simulink model "NCMS_AltMis_항공대"  (R2022a)
settings: Solver=FixedStepAuto  StartTime=0.0  StopTime=inf  FixedStep=SampleTime  RelTol=1e-3
InitFcn:
  | NCMS_AltMis_Init;
values from neighbouring files (symbols this model uses):
  Kdpr = 0.004    [NCMS_AltMis_Init_항공대.m]
  Kdrr = 0.004    [NCMS_AltMis_Init_항공대.m]
  Kdvz = 0.0254    [NCMS_AltMis_Init_항공대.m]
  Kdyr = 0.0298    [NCMS_AltMis_Init_항공대.m]
  Kipr = 0.1    [NCMS_AltMis_Init_항공대.m]
  Kirr = 0.1    [NCMS_AltMis_Init_항공대.m]
  Kivx = 0.0728/g    (= 0.00742099898063)    [NCMS_AltMis_Init_항공대.m]
  Kivy = 0.0728/g    (= 0.00742099898063)    [NCMS_AltMis_Init_항공대.m]
  Kivz = 0.6304    [NCMS_AltMis_Init_항공대.m]
  Kix = 0.02    [NCMS_AltMis_Init_항공대.m]
  Kiyaxis = 0.02    [NCMS_AltMis_Init_항공대.m]
  Kiyr = 0.7395    [NCMS_AltMis_Init_항공대.m]
  Kiz = 0.09    [NCMS_AltMis_Init_항공대.m]
  Kpp = 3.3894    [NCMS_AltMis_Init_항공대.m]
  Kppr = 0.1    [NCMS_AltMis_Init_항공대.m]
  Kpr = 3.3894    [NCMS_AltMis_Init_항공대.m]
  Kprr = 0.1    [NCMS_AltMis_Init_항공대.m]
  Kpvx = 2.1109/g    (= 0.215178389399)    [NCMS_AltMis_Init_항공대.m]
  Kpvy = 2.1109/g    (= 0.215178389399)    [NCMS_AltMis_Init_항공대.m]
  Kpvz = 0.3191    [NCMS_AltMis_Init_항공대.m]
  Kpx = 1    [NCMS_AltMis_Init_항공대.m]
  Kpy = 3.3894    [NCMS_AltMis_Init_항공대.m]
  Kpyaxis = 1    [NCMS_AltMis_Init_항공대.m]
  Kpyr = 0.3744    [NCMS_AltMis_Init_항공대.m]
  Kpz = 2.4    [NCMS_AltMis_Init_항공대.m]
  LAND_PRES_VEL = 0.2    [NCMS_AltMis_Init_항공대.m]
  MAX_CONTROL_ANGLE_PITCH = 30*pi/180    (= 0.523598775598)    [Init_FLIGHT_Hexacopter.m]    (also in NCMS_AltMis_Init_항공대.m = 0.349065850399)
  MAX_CONTROL_ANGLE_RATE_PITCH = 360*pi/180    (= 6.28318530718)    [Init_FLIGHT_Hexacopter.m]    (also in NCMS_AltMis_Init_항공대.m)
  MAX_CONTROL_ANGLE_RATE_ROLL = 360*pi/180    (= 6.28318530718)    [Init_FLIGHT_Hexacopter.m]    (also in NCMS_AltMis_Init_항공대.m)
  MAX_CONTROL_ANGLE_RATE_Y = 120*pi/180    (= 2.09439510239)    [Init_FLIGHT_Hexacopter.m]    (also in NCMS_AltMis_Init_항공대.m)
  MAX_CONTROL_ANGLE_ROLL = 30*pi/180    (= 0.523598775598)    [Init_FLIGHT_Hexacopter.m]    (also in NCMS_AltMis_Init_항공대.m = 0.349065850399)
  MAX_CONTROL_VELOCITY_XY = 1.5    [Init_FLIGHT_Hexacopter.m]    (also in NCMS_AltMis_Init_항공대.m)
  MAX_CONTROL_VELOCITY_Z = 1    [Init_FLIGHT_Hexacopter.m]    (also in NCMS_AltMis_Init_항공대.m)
  Npr = 50    [NCMS_AltMis_Init_항공대.m]
  Nrr = 50    [NCMS_AltMis_Init_항공대.m]
  Nvz = Npr    (= 50)    [NCMS_AltMis_Init_항공대.m]
  Nyr = 50    [NCMS_AltMis_Init_항공대.m]
  SampleTime = 1/250    (= 0.004)    [Init_FLIGHT_Hexacopter.m]    (also in NCMS_AltMis_Init_항공대.m = 0.01)
  THR_HOVER = 0.6085    [NCMS_AltMis_Init_항공대.m]
  THR_IDLE = 0.2    [NCMS_AltMis_Init_항공대.m]
undefined symbols (not defined in the file or in its folder): dev, Kdz, Main, Nz, pwm_output0
libraries: slpidlib x15, simulink x9, px4Sensorslib x3, px4uORBlib x3, uavalgslib x2, px4lib x1
(part 1 of 3)
settings Model: ExtModeTrigDuration=10  Creator=user  LastModifiedBy=ParkSeungWoo
settings SolverCC: PositivePriorityOrder=on
settings OptimizationCC: EnhancedBackFolding=on  PassReuseOutputArgsAs=Individual arguments  ZeroExternalMemoryAtStartup=off  ZeroInternalMemoryAtStartup=off  MaxStackSize=64  OptimizeBlockOrder=speed  DifferentSizesBufferReuse=on  OptimizationCustomize=off  EfficientTunableParamExpr=on
settings DebuggingCC: ParameterTunabilityLossMsg=error  UnconnectedInputMsg=warning  UnconnectedOutputMsg=warning  UnconnectedLineMsg=warning
settings HardwareCC: ProdBitPerPointer=32  ProdBitPerSizeT=32  ProdBitPerPtrDiffT=32  ProdLargestAtomicInteger=Long  ProdLargestAtomicFloat=Double  ProdWordSize=32  ProdLongLongMode=on  ProdHWDeviceType=ARM Compatible->ARM Cortex
settings SFSimCC: MATLABDynamicMemAlloc=off  SimTargetLang=C++
settings RTWCC: SystemTargetFile=ert.tlc  HardwareBoard=PX4 Pixhawk 4  TLCOptions="-aInlineSetEventsForThisBaseRateFcn=TLC_FALSE -aSuppressMultiTaskScheduler=TLC_FALSE  -aRateBasedStepFcn=0"  TemplateMakefile=ert_default_tmf  Toolchain=GNU Tools for PX4 Autopilots  TargetLang=C++  DLArmComputeVersion=19.05
settings CodeAppCC: ForceParamTrailComments=on  IgnoreCustomStorageClasses=off  OperatorAnnotations=on  SimulinkDataObjDesc=on  SFDataObjDesc=on  InsertBlockDesc=on
settings ERTTargetCC: MatFileLogging=on  ExtModeTransport=3  ExtModeStaticAlloc=on  ExtModeStaticAllocSize=1024  ExtModeMexFile=ext_xcp  ExtModeIntrfLevel=Level2 - Open

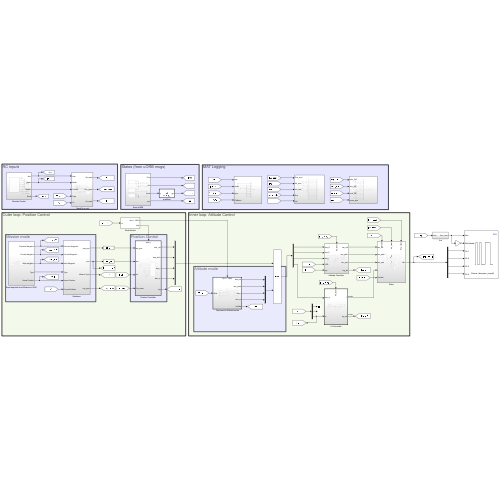
[thumbnail: Simulink's stored preview of the top-level diagram]
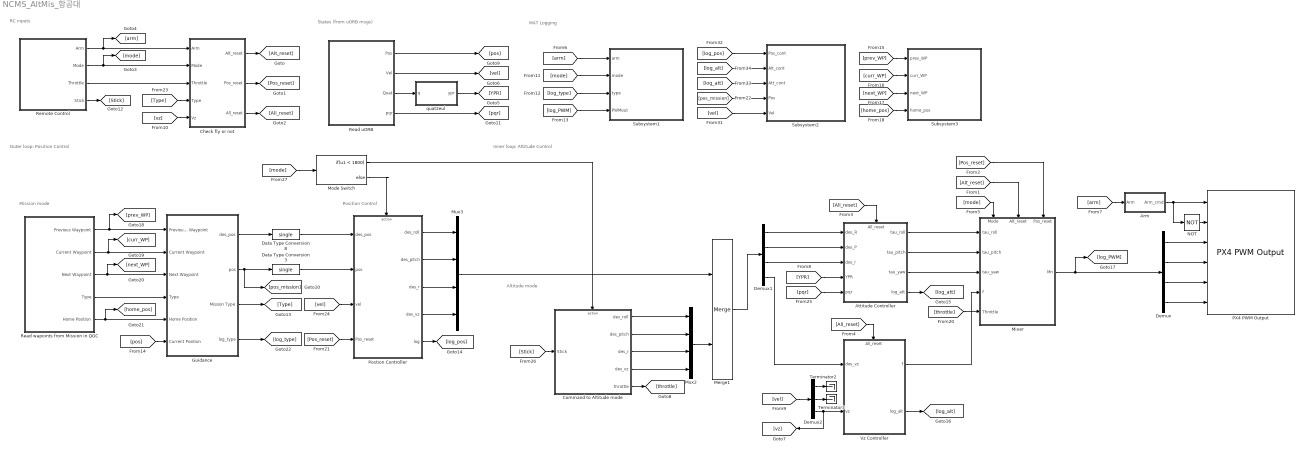
== system NCMS_AltMis_항공대 ==
  note: MAT Logging
  note: States (from uORB msgs)
  note: RC inputs
  note: Outer loop: Position Control
  note: Mission mode
  note: Inner loop: Attitude Control
  note: Altitude mode
  note: Position Control
  Arm : Subsystem
  Attitude Controller : Subsystem
      settings: PortSchema="{\"entries\":[{\"content\":{\"sides\":[{\"content\":{\"connectorIds\":[\"In1\",\"In2\",\"In3\",\"In4\",\"In5\"]},\"type\":\"ConnectorPlacement.EquallySpacedRectSide\",\"uuid\":\"77bb8164-b871-4593-8031-335c6110c17c\"},{\"content\":{\"connectorIds\":[\"Out1\",\"Out2\",\"Out3\",\"Out4\"],\"side\":\"RIGHT\"},\"type\":\"ConnectorPlacement.EquallySpacedRectSide\",\"uuid\":\"f99d9e85-7cc9-4d0a-ad5d-789571e28028\"},{\"content\":{\"connectorIds\":[\"In6\"],\"side\":\"TOP\"},\"type\":\"ConnectorPlacement.EquallySpacedRectSide\",\"uuid\":\"174eb658-0f52-43c7-ba1a-1a337b4835ca\"}]},\"type\":\"ConnectorPlacement.EquallySpacedConnector\",\"uuid\":\"7932b1f4-42ae-4dcf-8815-0888db42261d\"}],\"packageUris\":[\"http://schema.mathworks.com/mf0/Connector/R2020b\"],\"version\":\"1.0\"}"
  Check fly or not : Subsystem
  Command to Altitude mode : Subsystem  TreatAsAtomicUnit=on
  Data Type Conversion3 : DataTypeConversion  OutDataTypeStr=single  SaturateOnIntegerOverflow=off  RndMeth=Floor
  Data Type Conversion8 : DataTypeConversion  OutDataTypeStr=single  SaturateOnIntegerOverflow=off  RndMeth=Floor
  Demux : Demux
  Demux1 : Demux
  Demux2 : Demux  Outputs=3
  Guidance : Subsystem
  Merge1 : Merge
  Mixer : Subsystem
      settings: PortSchema="{\"entries\":[{\"content\":{\"sides\":[{\"content\":{\"connectorIds\":[\"In1\",\"In2\",\"In3\",\"In4\",\"In5\"]},\"type\":\"ConnectorPlacement.EquallySpacedRectSide\",\"uuid\":\"058a1e3b-c324-4fa3-8465-0a7a3d8b0c1a\"},{\"content\":{\"connectorIds\":[\"Out1\"],\"side\":\"RIGHT\"},\"type\":\"ConnectorPlacement.EquallySpacedRectSide\",\"uuid\":\"ff1c26dd-92d4-4453-a7b4-224d07c62cb4\"},{\"content\":{\"connectorIds\":[\"In6\",\"In7\",\"In8\"],\"side\":\"TOP\"},\"type\":\"ConnectorPlacement.EquallySpacedRectSide\",\"uuid\":\"9bc4c9d9-536a-4d54-a641-00bc48245afe\"}]},\"type\":\"ConnectorPlacement.EquallySpacedConnector\",\"uuid\":\"86048a90-d386-4461-986e-b57c6ef8ec17\"}],\"packageUris\":[\"http://schema.mathworks.com/mf0/Connector/R2020b\"],\"version\":\"1.0\"}"
  Mode Switch : If  IfExpression=u1 < 1800
  Mux2 : Mux
  Mux3 : Mux
  NOT : Logic  Operator=NOT  IconShape=distinctive  AllPortsSameDT=off  OutDataTypeStr=boolean
  PX4 PWM Output : px4lib/PX4 PWM Output  pwmDevice=Main (/dev/pwm_output0)  pwmChannel1_=on  pwmChannel2_=on  pwmChannel3_=on  pwmChannel4_=on  pwmChannel5_=off  pwmChannel6_=off  pwmChannel7_=off  pwmChannel8_=off  forceTerminateFailsafe=off  outputErrorStatus=off
      settings: SourceProductBaseCode=PX4AUTOPILOTS
  Postion Controller : Subsystem
  Read uORB : Subsystem
  Read wapoints from Mission in QGC : Subsystem
  Remote Control : Subsystem
  Subsystem1 : Subsystem
  Subsystem2 : Subsystem
  Subsystem3 : Subsystem
  Terminator2 : Terminator
  Terminator3 : Terminator
  Vz Controller : Subsystem  TreatAsAtomicUnit=on
      settings: PortSchema="{\"entries\":[{\"content\":{\"sides\":[{\"content\":{\"connectorIds\":[\"In1\",\"In2\"]},\"type\":\"ConnectorPlacement.EquallySpacedRectSide\",\"uuid\":\"343d190f-1f89-45cd-8068-8c2f27ac01d9\"},{\"content\":{\"connectorIds\":[\"Out1\",\"Out2\"],\"side\":\"RIGHT\"},\"type\":\"ConnectorPlacement.EquallySpacedRectSide\",\"uuid\":\"f56c4d57-5cdb-41f3-bf2e-c6d595243432\"},{\"content\":{\"connectorIds\":[\"In3\"],\"side\":\"TOP\"},\"type\":\"ConnectorPlacement.EquallySpacedRectSide\",\"uuid\":\"16744f99-c08a-4b46-9015-9ea58d319995\"}]},\"type\":\"ConnectorPlacement.EquallySpacedConnector\",\"uuid\":\"48685039-fe1b-4520-bbd0-43ddf02d7910\"}],\"packageUris\":[\"http://schema.mathworks.com/mf0/Connector/R2020b\"],\"version\":\"1.0\"}"
  quat2eul : MATLAB Function  TreatAsAtomicUnit=on
  wires:
  Demux/1 -> PX4 PWM Output/3
  Demux/2 -> PX4 PWM Output/4
  Demux/3 -> PX4 PWM Output/5
  Demux/4 -> PX4 PWM Output/6
  NOT/1 -> PX4 PWM Output/2
  Read uORB/3(Quat) -> quat2eul/1(q)
  Demux1/1 -> Attitude Controller/1(des_R)
  Demux1/2 -> Attitude Controller/2(des_P)
  Attitude Controller/1(tau_roll) -> Mixer/1(tau_roll)
  Attitude Controller/2(tau_pitch) -> Mixer/2(tau_pitch)
  Arm/1(Arm_cmd) -> NOT/1, PX4 PWM Output/1
  Demux1/3 -> Attitude Controller/3(des_r)
  Attitude Controller/3(tau_yaw) -> Mixer/3(tau_yaw)
  Demux2/2 -> Terminator3/1
  Demux2/1 -> Terminator2/1
  Vz Controller/1(f) -> Mixer/4(f)
  Demux2/3 -> Vz Controller/2(vz), [vz]
  Read uORB/2(Vel) -> [vel]
  Demux1/4 -> Vz Controller/1(des_vz)
  Mux2/1 -> Merge1/2
  Command to Altitude mode/3(des_r) -> Mux2/3
  Command to Altitude mode/2(des_pitch) -> Mux2/2
  Command to Altitude mode/1(des_roll) -> Mux2/1
  Command to Altitude mode/4(des_vz) -> Mux2/4
  Remote Control/4(Stick) -> [Stick]
  Postion Controller/2(des_pitch) -> Mux3/2
  Postion Controller/3(des_r) -> Mux3/3
  Postion Controller/1(des_roll) -> Mux3/1
  Mux3/1 -> Merge1/1
  Remote Control/2(Mode) -> [mode], Check fly or not/2(Mode)
  Remote Control/1(Arm) -> [arm], Check fly or not/1(Arm)
  Guidance/1(des_pos) -> Data Type Conversion8/1
  Read uORB/1(Pos) -> [pos]
  Postion Controller/4(des_vz) -> Mux3/4
  Data Type Conversion8/1 -> Postion Controller/1(des_pos)
  Data Type Conversion3/1 -> Postion Controller/2(pos)
  Merge1/1 -> Demux1/1
  Guidance/3(Mission Type) -> [Type]
  Check fly or not/1(Alt_reset) -> [Alt_reset]
  [Alt_reset] -> Mixer/7(Alt_reset)
  Check fly or not/2(Pos_reset) -> [Pos_reset]
  [Pos_reset] -> Mixer/8(Pos_reset)
  Check fly or not/3(All_reset) -> [All_reset]
  [All_reset] -> Attitude Controller/6(All_reset)
  [All_reset] -> Vz Controller/3(All_reset)
  [mode] -> Mixer/6(Mode)
  [arm] -> Arm/1(Arm)
  quat2eul/1(ypr) -> [YPR]
  [YPR] -> Attitude Controller/4(YPR)
  [vel] -> Demux2/1
  [vz] -> Check fly or not/5(Vz)
  [throttle] -> Mixer/5(Throttle)
  Command to Altitude mode/5(throttle) -> [throttle]
  [Pos_reset] -> Postion Controller/4(Pos_reset)
  Guidance/2(pos) -> [pos_mission], Data Type Conversion3/1
  [Type] -> Check fly or not/4(Type)
  Mode Switch/2 -> Postion Controller/Action
  Mode Switch/1 -> Command to Altitude mode/Action
  [vel] -> Postion Controller/3(vel)
  Read uORB/4(pqr) -> [pqr]
  [Stick] -> Command to Altitude mode/1(Stick)
  Remote Control/3(Throttle) -> Check fly or not/3(Throttle)
  [mode] -> Mode Switch/1
  Postion Controller/5(log) -> [log_pos]
  Attitude Controller/4(log_att) -> [log_att]
  Vz Controller/2(log_alt) -> [log_alt]
  Mixer/1(Mn) -> [log_PWM], Demux/1
  [arm] -> Subsystem1/1(arm)
  [mode] -> Subsystem1/2(mode)
  [log_type] -> Subsystem1/3(type)
  [log_PWM] -> Subsystem1/4(PWMout)
  [pos] -> Guidance/6(Current Position)
  Read wapoints from Mission in QGC/2(Current Waypoint) -> [curr_WP], Guidance/2(Current Waypoint)
  Read wapoints from Mission in QGC/3(Next Waypoint) -> [next_WP], Guidance/3(Next Waypoint)
  Read wapoints from Mission in QGC/4(Type) -> Guidance/4(Type)
  Read wapoints from Mission in QGC/5(Home Position) -> [home_pos], Guidance/5(Home Position)
  [pqr] -> Attitude Controller/5(pqr)
  [vel] -> Subsystem2/5(Vel)
  [pos_mission] -> Subsystem2/4(Pos)
  [log_att] -> Subsystem2/3(Att_cont)
  [log_alt] -> Subsystem2/2(Alt_cont)
  [log_pos] -> Subsystem2/1(Pos_cont)
  [home_pos] -> Subsystem3/4(home_pos)
  [next_WP] -> Subsystem3/3(next_WP)
  [curr_WP] -> Subsystem3/2(curr_WP)
  [prev_WP] -> Subsystem3/1(prev_WP)
  Guidance/4(log_type) -> [log_type]
  Read wapoints from Mission in QGC/1(Previous Waypoint) -> [prev_WP], Guidance/1(Previous Waypoint)

== system NCMS_AltMis_항공대/Arm ==
  Arm : Inport
  Compare To Constant3 : simulink/Logic and Bit Operations/Compare To Constant  relop=>=  const=uint16(1800)  OutDataTypeStr=boolean
  Arm_cmd : Outport  VectorParamsAs1DForOutWhenUnconnected=off
  wires:
  Arm/1 -> Compare To Constant3/1
  Compare To Constant3/1 -> Arm_cmd/1

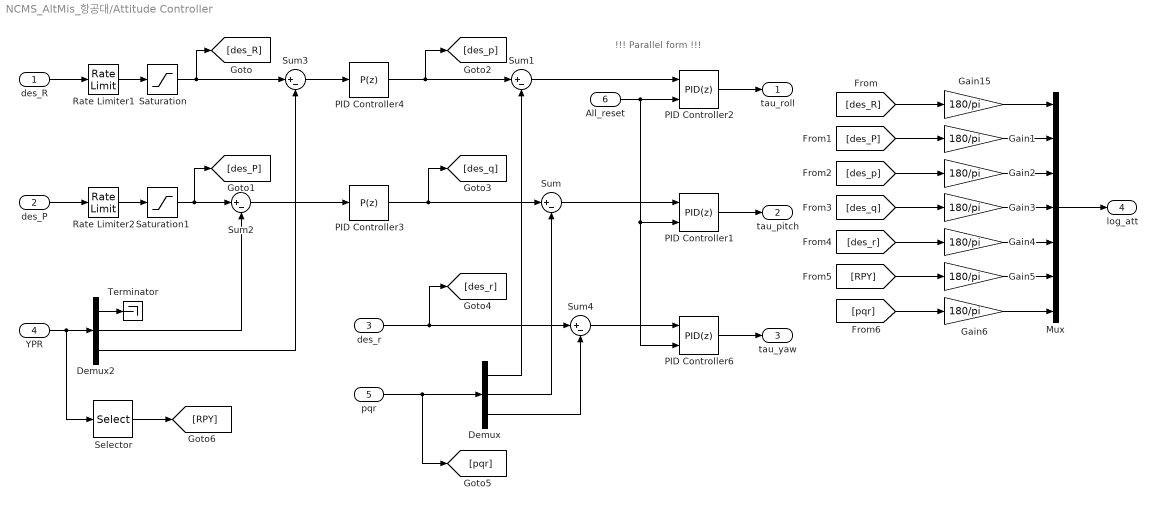
== system NCMS_AltMis_항공대/Attitude Controller ==
  note: !!! Parallel form !!!
  des_R : Inport
  des_P : Inport  Port=2
  des_r : Inport  Port=3
  YPR : Inport  Port=4
  pqr : Inport  Port=5
  All_reset : Inport  Port=6
  Demux : Demux  Outputs=3
  Demux2 : Demux  Outputs=3
  Gain{1..6,15} (7 alike) : Gain  Gain=180/pi
  Mux : Mux  Inputs=7
  PID Controller1 : slpidlib/PID Controller  Controller=PID  Form=Parallel  TimeDomain=Discrete-time  UseExternalTs=off  SampleTime=SampleTime  IntegratorMethod=Forward Euler  FilterMethod=Forward Euler  ControllerParametersSource=internal  P=Kppr  I=Kipr  UseKiTs=off  D=Kdpr  N=Npr  UseFilter=on  TunerSelectOption=Transfer Function Based (PID Tuner App)  InitialConditionSource=internal  InitialConditionForIntegrator=0  InitialConditionForFilter=0  DifferentiatorICPrevScaledInput=0  ExternalReset=either  TrackingMode=off  Kt=1  LimitOutput=on  SatLimitsSource=internal  UpperSaturationLimit=0.2  LowerSaturationLimit=-0.2  LinearizeAsGain=on  AntiWindupMode=clamping  Kb=1  POutMin=[]  POutMax=[]  IOutMin=[]  IOutMax=[]  DOutMin=[]  DOutMax=[]  NOutMin=[]  NOutMax=[]  SumOutMin=[]  SumOutMax=[]  SaturationOutMin=[]  SaturationOutMax=[]  PParamMin=[]  PParamMax=[]  IParamMin=[]  IParamMax=[]  DParamMin=[]  DParamMax=[]  NParamMin=[]  NParamMax=[]  KbParamMin=[]  KbParamMax=[]  KtParamMin=[]  KtParamMax=[]  KbOutMin=[]  KbOutMax=[]  KtOutMin=[]  KtOutMax=[]  IntegratorOutMin=[]  IntegratorOutMax=[]  FilterOutMin=[]  FilterOutMax=[]  SumI1OutMin=[]  SumI1OutMax=[]  SumI2OutMin=[]  SumI2OutMax=[]  SumI3OutMin=[]  SumI3OutMax=[]  SumI4OutMin=[]  SumI4OutMax=[]  SumDOutMin=[]  SumDOutMax=[]  DifferentiatorOutMin=[]  DifferentiatorOutMax=[]  FilterDiffOutCoefMin=[]  FilterDiffOutCoefMax=[]  ReciprocalOutMin=[]  ReciprocalOutMax=[]  SumDenOutMin=[]  SumDenOutMax=[]  SumNumOutMin=[]  SumNumOutMax=[]  DivideOutMin=[]  DivideOutMax=[]  UdiffTsProdOutMin=[]  UdiffTsProdOutMax=[]  NTsProdOutMin=[]  NTsProdOutMax=[]  UintegralTsProdOutMin=[]  UintegralTsProdOutMax=[]  UngainTsProdOutMin=[]  UngainTsProdOutMax=[]  IntegratorContinuousStateAttributes=''  IntegratorStateMustResolveToSignalObject=off  IntegratorRTWStateStorageClass=Auto  FilterContinuousStateAttributes=''  FilterStateMustResolveToSignalObject=off  FilterRTWStateStorageClass=Auto  ParallelPVariant=InternalParameters  IdealPVariant=Disabled  IVariant=InternalParameters  DVariant=InternalParameters  IntegratorVariant=Discrete  SatVariant=Enabled  AWVariant=DiscClampingParallel  PCopyVariant=Disabled  TRVariant=Disabled  FdbkBlocksVariant=Forward  IdealPFdbkVariant=Disabled  SatFdbkVariant=Disabled  DerivativeFilterVariant=ForwardEulerFilter  NVariant=InternalParameters  NCopyVariant=Disabled  FilterICVariant=InternalICsFilter  IntegratorICVariant=InternalICs  ExternalResetVariant=ExternalReset  TRSumVariant=Passthrough  SumFdbkVariant=Disabled  SumVariant=Sum_PID  TsampFilterVariant=InternalTs  TsampNgainVariant=Passthrough  TsampIntegralVariant=Passthrough  ExternalSaturationOutDataTypeStr=Inherit: Same as second input  aMode=0
  PID Controller2 : slpidlib/PID Controller  Controller=PID  Form=Parallel  TimeDomain=Discrete-time  UseExternalTs=off  SampleTime=SampleTime  IntegratorMethod=Forward Euler  FilterMethod=Forward Euler  ControllerParametersSource=internal  P=Kprr  I=Kirr  UseKiTs=off  D=Kdrr  N=Nrr  UseFilter=on  TunerSelectOption=Transfer Function Based (PID Tuner App)  InitialConditionSource=internal  InitialConditionForIntegrator=0  InitialConditionForFilter=0  DifferentiatorICPrevScaledInput=0  ExternalReset=either  TrackingMode=off  Kt=1  LimitOutput=on  SatLimitsSource=internal  UpperSaturationLimit=0.2  LowerSaturationLimit=-0.2  LinearizeAsGain=on  AntiWindupMode=clamping  Kb=1  POutMin=[]  POutMax=[]  IOutMin=[]  IOutMax=[]  DOutMin=[]  DOutMax=[]  NOutMin=[]  NOutMax=[]  SumOutMin=[]  SumOutMax=[]  SaturationOutMin=[]  SaturationOutMax=[]  PParamMin=[]  PParamMax=[]  IParamMin=[]  IParamMax=[]  DParamMin=[]  DParamMax=[]  NParamMin=[]  NParamMax=[]  KbParamMin=[]  KbParamMax=[]  KtParamMin=[]  KtParamMax=[]  KbOutMin=[]  KbOutMax=[]  KtOutMin=[]  KtOutMax=[]  IntegratorOutMin=[]  IntegratorOutMax=[]  FilterOutMin=[]  FilterOutMax=[]  SumI1OutMin=[]  SumI1OutMax=[]  SumI2OutMin=[]  SumI2OutMax=[]  SumI3OutMin=[]  SumI3OutMax=[]  SumI4OutMin=[]  SumI4OutMax=[]  SumDOutMin=[]  SumDOutMax=[]  DifferentiatorOutMin=[]  DifferentiatorOutMax=[]  FilterDiffOutCoefMin=[]  FilterDiffOutCoefMax=[]  ReciprocalOutMin=[]  ReciprocalOutMax=[]  SumDenOutMin=[]  SumDenOutMax=[]  SumNumOutMin=[]  SumNumOutMax=[]  DivideOutMin=[]  DivideOutMax=[]  UdiffTsProdOutMin=[]  UdiffTsProdOutMax=[]  NTsProdOutMin=[]  NTsProdOutMax=[]  UintegralTsProdOutMin=[]  UintegralTsProdOutMax=[]  UngainTsProdOutMin=[]  UngainTsProdOutMax=[]  IntegratorContinuousStateAttributes=''  IntegratorStateMustResolveToSignalObject=off  IntegratorRTWStateStorageClass=Auto  FilterContinuousStateAttributes=''  FilterStateMustResolveToSignalObject=off  FilterRTWStateStorageClass=Auto  ParallelPVariant=InternalParameters  IdealPVariant=Disabled  IVariant=InternalParameters  DVariant=InternalParameters  IntegratorVariant=Discrete  SatVariant=Enabled  AWVariant=DiscClampingParallel  PCopyVariant=Disabled  TRVariant=Disabled  FdbkBlocksVariant=Forward  IdealPFdbkVariant=Disabled  SatFdbkVariant=Disabled  DerivativeFilterVariant=ForwardEulerFilter  NVariant=InternalParameters  NCopyVariant=Disabled  FilterICVariant=InternalICsFilter  IntegratorICVariant=InternalICs  ExternalResetVariant=ExternalReset  TRSumVariant=Passthrough  SumFdbkVariant=Disabled  SumVariant=Sum_PID  TsampFilterVariant=InternalTs  TsampNgainVariant=Passthrough  TsampIntegralVariant=Passthrough  ExternalSaturationOutDataTypeStr=Inherit: Same as second input  aMode=0
  PID Controller3 : slpidlib/PID Controller  Controller=P  Form=Parallel  TimeDomain=Discrete-time  UseExternalTs=off  SampleTime=SampleTime  IntegratorMethod=Forward Euler  FilterMethod=Forward Euler  ControllerParametersSource=internal  P=Kpp  I=1  UseKiTs=off  D=0  N=100  UseFilter=on  TunerSelectOption=Transfer Function Based (PID Tuner App)  InitialConditionSource=internal  InitialConditionForIntegrator=0  InitialConditionForFilter=0  DifferentiatorICPrevScaledInput=0  ExternalReset=none  TrackingMode=off  Kt=1  LimitOutput=on  SatLimitsSource=internal  UpperSaturationLimit=MAX_CONTROL_ANGLE_RATE_PITCH  LowerSaturationLimit=-MAX_CONTROL_ANGLE_RATE_PITCH  LinearizeAsGain=on  AntiWindupMode=none  Kb=1  POutMin=[]  POutMax=[]  IOutMin=[]  IOutMax=[]  DOutMin=[]  DOutMax=[]  NOutMin=[]  NOutMax=[]  SumOutMin=[]  SumOutMax=[]  SaturationOutMin=[]  SaturationOutMax=[]  PParamMin=[]  PParamMax=[]  IParamMin=[]  IParamMax=[]  DParamMin=[]  DParamMax=[]  NParamMin=[]  NParamMax=[]  KbParamMin=[]  KbParamMax=[]  KtParamMin=[]  KtParamMax=[]  KbOutMin=[]  KbOutMax=[]  KtOutMin=[]  KtOutMax=[]  IntegratorOutMin=[]  IntegratorOutMax=[]  FilterOutMin=[]  FilterOutMax=[]  SumI1OutMin=[]  SumI1OutMax=[]  SumI2OutMin=[]  SumI2OutMax=[]  SumI3OutMin=[]  SumI3OutMax=[]  SumI4OutMin=[]  SumI4OutMax=[]  SumDOutMin=[]  SumDOutMax=[]  DifferentiatorOutMin=[]  DifferentiatorOutMax=[]  FilterDiffOutCoefMin=[]  FilterDiffOutCoefMax=[]  ReciprocalOutMin=[]  ReciprocalOutMax=[]  SumDenOutMin=[]  SumDenOutMax=[]  SumNumOutMin=[]  SumNumOutMax=[]  DivideOutMin=[]  DivideOutMax=[]  UdiffTsProdOutMin=[]  UdiffTsProdOutMax=[]  NTsProdOutMin=[]  NTsProdOutMax=[]  UintegralTsProdOutMin=[]  UintegralTsProdOutMax=[]  UngainTsProdOutMin=[]  UngainTsProdOutMax=[]  IntegratorContinuousStateAttributes=''  IntegratorStateMustResolveToSignalObject=off  IntegratorRTWStateStorageClass=Auto  FilterContinuousStateAttributes=''  FilterStateMustResolveToSignalObject=off  FilterRTWStateStorageClass=Auto  ParallelPVariant=InternalParameters  IdealPVariant=Disabled  IVariant=Disabled  DVariant=Disabled  IntegratorVariant=Disabled  SatVariant=Enabled  AWVariant=Disabled  PCopyVariant=Disabled  TRVariant=Disabled  FdbkBlocksVariant=Forward  IdealPFdbkVariant=Disabled  SatFdbkVariant=Disabled  DerivativeFilterVariant=Disabled  NVariant=Disabled  NCopyVariant=Disabled_SignalSpec  FilterICVariant=Disabled  IntegratorICVariant=Disabled  ExternalResetVariant=Disabled  TRSumVariant=Passthrough  SumFdbkVariant=Disabled  SumVariant=Passthrough_P  TsampFilterVariant=InternalTs  TsampNgainVariant=Passthrough  TsampIntegralVariant=Disabled_SignalSpec  ExternalSaturationOutDataTypeStr=Inherit: Same as second input  aMode=0
  PID Controller4 : slpidlib/PID Controller  Controller=P  Form=Parallel  TimeDomain=Discrete-time  UseExternalTs=off  SampleTime=SampleTime  IntegratorMethod=Forward Euler  FilterMethod=Forward Euler  ControllerParametersSource=internal  P=Kpr  I=1  UseKiTs=off  D=0  N=100  UseFilter=on  TunerSelectOption=Transfer Function Based (PID Tuner App)  InitialConditionSource=internal  InitialConditionForIntegrator=0  InitialConditionForFilter=0  DifferentiatorICPrevScaledInput=0  ExternalReset=none  TrackingMode=off  Kt=1  LimitOutput=on  SatLimitsSource=internal  UpperSaturationLimit=MAX_CONTROL_ANGLE_RATE_ROLL  LowerSaturationLimit=-MAX_CONTROL_ANGLE_RATE_ROLL  LinearizeAsGain=on  AntiWindupMode=none  Kb=1  POutMin=[]  POutMax=[]  IOutMin=[]  IOutMax=[]  DOutMin=[]  DOutMax=[]  NOutMin=[]  NOutMax=[]  SumOutMin=[]  SumOutMax=[]  SaturationOutMin=[]  SaturationOutMax=[]  PParamMin=[]  PParamMax=[]  IParamMin=[]  IParamMax=[]  DParamMin=[]  DParamMax=[]  NParamMin=[]  NParamMax=[]  KbParamMin=[]  KbParamMax=[]  KtParamMin=[]  KtParamMax=[]  KbOutMin=[]  KbOutMax=[]  KtOutMin=[]  KtOutMax=[]  IntegratorOutMin=[]  IntegratorOutMax=[]  FilterOutMin=[]  FilterOutMax=[]  SumI1OutMin=[]  SumI1OutMax=[]  SumI2OutMin=[]  SumI2OutMax=[]  SumI3OutMin=[]  SumI3OutMax=[]  SumI4OutMin=[]  SumI4OutMax=[]  SumDOutMin=[]  SumDOutMax=[]  DifferentiatorOutMin=[]  DifferentiatorOutMax=[]  FilterDiffOutCoefMin=[]  FilterDiffOutCoefMax=[]  ReciprocalOutMin=[]  ReciprocalOutMax=[]  SumDenOutMin=[]  SumDenOutMax=[]  SumNumOutMin=[]  SumNumOutMax=[]  DivideOutMin=[]  DivideOutMax=[]  UdiffTsProdOutMin=[]  UdiffTsProdOutMax=[]  NTsProdOutMin=[]  NTsProdOutMax=[]  UintegralTsProdOutMin=[]  UintegralTsProdOutMax=[]  UngainTsProdOutMin=[]  UngainTsProdOutMax=[]  IntegratorContinuousStateAttributes=''  IntegratorStateMustResolveToSignalObject=off  IntegratorRTWStateStorageClass=Auto  FilterContinuousStateAttributes=''  FilterStateMustResolveToSignalObject=off  FilterRTWStateStorageClass=Auto  ParallelPVariant=InternalParameters  IdealPVariant=Disabled  IVariant=Disabled  DVariant=Disabled  IntegratorVariant=Disabled  SatVariant=Enabled  AWVariant=Disabled  PCopyVariant=Disabled  TRVariant=Disabled  FdbkBlocksVariant=Forward  IdealPFdbkVariant=Disabled  SatFdbkVariant=Disabled  DerivativeFilterVariant=Disabled  NVariant=Disabled  NCopyVariant=Disabled_SignalSpec  FilterICVariant=Disabled  IntegratorICVariant=Disabled  ExternalResetVariant=Disabled  TRSumVariant=Passthrough  SumFdbkVariant=Disabled  SumVariant=Passthrough_P  TsampFilterVariant=InternalTs  TsampNgainVariant=Passthrough  TsampIntegralVariant=Disabled_SignalSpec  ExternalSaturationOutDataTypeStr=Inherit: Same as second input  aMode=0
  PID Controller6 : slpidlib/PID Controller  Controller=PID  Form=Parallel  TimeDomain=Discrete-time  UseExternalTs=off  SampleTime=SampleTime  IntegratorMethod=Forward Euler  FilterMethod=Forward Euler  ControllerParametersSource=internal  P=Kpyr  I=Kiyr  UseKiTs=off  D=Kdyr  N=Nyr  UseFilter=on  TunerSelectOption=Transfer Function Based (PID Tuner App)  InitialConditionSource=internal  InitialConditionForIntegrator=0  InitialConditionForFilter=0  DifferentiatorICPrevScaledInput=0  ExternalReset=either  TrackingMode=off  Kt=1  LimitOutput=on  SatLimitsSource=internal  UpperSaturationLimit=0.4  LowerSaturationLimit=-0.4  LinearizeAsGain=on  AntiWindupMode=clamping  Kb=1  POutMin=[]  POutMax=[]  IOutMin=[]  IOutMax=[]  DOutMin=[]  DOutMax=[]  NOutMin=[]  NOutMax=[]  SumOutMin=[]  SumOutMax=[]  SaturationOutMin=[]  SaturationOutMax=[]  PParamMin=[]  PParamMax=[]  IParamMin=[]  IParamMax=[]  DParamMin=[]  DParamMax=[]  NParamMin=[]  NParamMax=[]  KbParamMin=[]  KbParamMax=[]  KtParamMin=[]  KtParamMax=[]  KbOutMin=[]  KbOutMax=[]  KtOutMin=[]  KtOutMax=[]  IntegratorOutMin=[]  IntegratorOutMax=[]  FilterOutMin=[]  FilterOutMax=[]  SumI1OutMin=[]  SumI1OutMax=[]  SumI2OutMin=[]  SumI2OutMax=[]  SumI3OutMin=[]  SumI3OutMax=[]  SumI4OutMin=[]  SumI4OutMax=[]  SumDOutMin=[]  SumDOutMax=[]  DifferentiatorOutMin=[]  DifferentiatorOutMax=[]  FilterDiffOutCoefMin=[]  FilterDiffOutCoefMax=[]  ReciprocalOutMin=[]  ReciprocalOutMax=[]  SumDenOutMin=[]  SumDenOutMax=[]  SumNumOutMin=[]  SumNumOutMax=[]  DivideOutMin=[]  DivideOutMax=[]  UdiffTsProdOutMin=[]  UdiffTsProdOutMax=[]  NTsProdOutMin=[]  NTsProdOutMax=[]  UintegralTsProdOutMin=[]  UintegralTsProdOutMax=[]  UngainTsProdOutMin=[]  UngainTsProdOutMax=[]  IntegratorContinuousStateAttributes=''  IntegratorStateMustResolveToSignalObject=off  IntegratorRTWStateStorageClass=Auto  FilterContinuousStateAttributes=''  FilterStateMustResolveToSignalObject=off  FilterRTWStateStorageClass=Auto  ParallelPVariant=InternalParameters  IdealPVariant=Disabled  IVariant=InternalParameters  DVariant=InternalParameters  IntegratorVariant=Discrete  SatVariant=Enabled  AWVariant=DiscClampingParallel  PCopyVariant=Disabled  TRVariant=Disabled  FdbkBlocksVariant=Forward  IdealPFdbkVariant=Disabled  SatFdbkVariant=Disabled  DerivativeFilterVariant=ForwardEulerFilter  NVariant=InternalParameters  NCopyVariant=Disabled  FilterICVariant=InternalICsFilter  IntegratorICVariant=InternalICs  ExternalResetVariant=ExternalReset  TRSumVariant=Passthrough  SumFdbkVariant=Disabled  SumVariant=Sum_PID  TsampFilterVariant=InternalTs  TsampNgainVariant=Passthrough  TsampIntegralVariant=Passthrough  ExternalSaturationOutDataTypeStr=Inherit: Same as second input  aMode=0
  Rate Limiter1 : RateLimiter  RisingSlewLimit=40*pi/180  FallingSlewLimit=-40*pi/180  SampleTimeMode=inherited
  Rate Limiter2 : RateLimiter  RisingSlewLimit=40*pi/180  FallingSlewLimit=-40*pi/180  SampleTimeMode=inherited
  Saturation : Saturate  UpperLimit=MAX_CONTROL_ANGLE_ROLL  LowerLimit=-MAX_CONTROL_ANGLE_ROLL
  Saturation1 : Saturate  UpperLimit=MAX_CONTROL_ANGLE_PITCH  LowerLimit=-MAX_CONTROL_ANGLE_PITCH
  Selector : Selector  InputPortWidth=3  IndexOptions=Index vector (dialog)  Indices=[3 2 1]  OutputSizes=1
  Sum{,1..4} (5 alike) : Sum  Inputs=|+-
  Terminator : Terminator
  tau_roll : Outport
  tau_pitch : Outport  Port=2
  tau_yaw : Outport  Port=3
  log_att : Outport  Port=4
  wires:
  Rate Limiter2/1 -> Saturation1/1
  PID Controller6/1 -> tau_yaw/1
  [des_r] -> Gain4/1
  Gain4/1 -> Mux/5
  Gain3/1 -> Mux/4
  Demux2/2 -> Sum2/2
  Gain6/1 -> Mux/7
  PID Controller3/1 -> [des_q], Sum/1
  [des_q] -> Gain3/1
  [pqr] -> Gain6/1
  Demux2/3 -> Sum3/2
  PID Controller2/1 -> tau_roll/1
  [des_p] -> Gain2/1
  Gain2/1 -> Mux/3
  Mux/1 -> log_att/1
  Sum2/1 -> PID Controller3/1
  Gain15/1 -> Mux/1
  PID Controller1/1 -> tau_pitch/1
  Gain1/1 -> Mux/2
  des_r/1 -> [des_r], Sum4/1
  Sum4/1 -> PID Controller6/1
  All_reset/1 -> PID Controller2/2, PID Controller6/2, PID Controller1/2
  Demux/3 -> Sum4/2
  PID Controller4/1 -> [des_p], Sum1/1
  Demux2/1 -> Terminator/1
  Sum/1 -> PID Controller1/1
  [RPY] -> Gain5/1
  Demux/2 -> Sum/2
  YPR/1 -> Selector/1, Demux2/1
  [des_R] -> Gain15/1
  des_P/1 -> Rate Limiter2/1
  [des_P] -> Gain1/1
  Saturation1/1 -> [des_P], Sum2/1
  Demux/1 -> Sum1/2
  Saturation/1 -> [des_R], Sum3/1
  Sum3/1 -> PID Controller4/1
  Selector/1 -> [RPY]
  Rate Limiter1/1 -> Saturation/1
  pqr/1 -> [pqr], Demux/1
  des_R/1 -> Rate Limiter1/1
  Sum1/1 -> PID Controller2/1
  Gain5/1 -> Mux/6

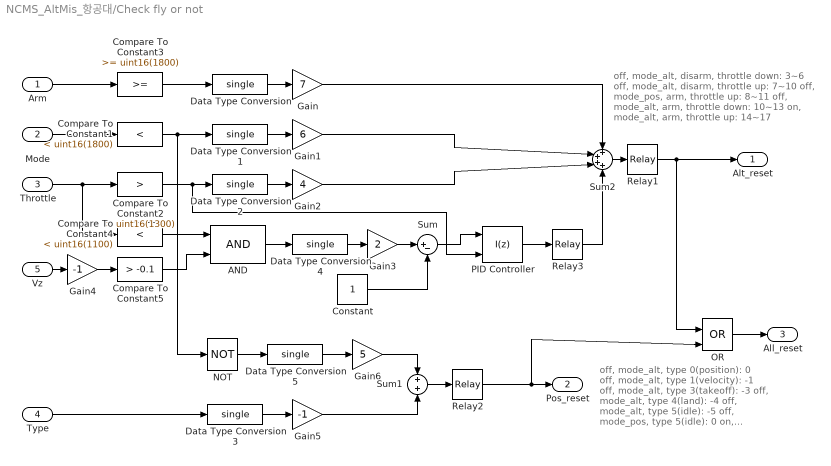
== system NCMS_AltMis_항공대/Check fly or not ==
  note: off, mode_alt, disarm, throttle down: 3~6
      | off, mode_alt, disarm, throttle up: 7~10
      | off, mode_pos, arm, throttle up: 8~11
      | off, mode_alt, arm, throttle down: 10~13
      | on, mode_alt, arm, throttle up: 14~17
  note: off, mode_alt, type 0(position): 0
      | off, mode_alt, type 1(velocity): -1
      | off, mode_alt, type 3(takeoff): -3
      | off, mode_alt, type 4(land): -4
      | off, mode_alt, type 5(idle): -5
      | off, mode_pos, type 5(idle): 0
      | on, mode_pos, type 0(position): 5
      | on, mode_pos, type 1(velocity): 4
      | on, mode_pos, type 3(takeoff): 2
      | on, mode_pos, type 4(land): 1
  Arm : Inport
  Mode : Inport  Port=2
  Throttle : Inport  Port=3
  Type : Inport  Port=4
  Vz : Inport  Port=5
  AND : Logic  IconShape=distinctive  AllPortsSameDT=off  OutDataTypeStr=boolean
  Compare To Constant1 : simulink/Logic and Bit Operations/Compare To Constant  relop=<  const=uint16(1800)  OutDataTypeStr=boolean
  Compare To Constant2 : simulink/Logic and Bit Operations/Compare To Constant  relop=>  const=uint16(1300)  OutDataTypeStr=boolean
  Compare To Constant3 : simulink/Logic and Bit Operations/Compare To Constant  relop=>=  const=uint16(1800)  OutDataTypeStr=boolean
  Compare To Constant4 : simulink/Logic and Bit Operations/Compare To Constant  relop=<  const=uint16(1100)  OutDataTypeStr=boolean
  Compare To Constant5 : simulink/Logic and Bit Operations/Compare To Constant  relop=>  const=-0.1  OutDataTypeStr=boolean
  Constant : Constant  OutDataTypeStr=single
  Data Type Conversion{,1..5} (6 alike) : DataTypeConversion  OutDataTypeStr=single  SaturateOnIntegerOverflow=off  RndMeth=Floor
  Gain : Gain  Gain=7
  Gain1 : Gain  Gain=6
  Gain2 : Gain  Gain=4
  Gain3 : Gain  Gain=2
  Gain4 : Gain  Gain=-1
  Gain5 : Gain  Gain=-1
  Gain6 : Gain  Gain=5
  NOT : Logic  Operator=NOT  IconShape=distinctive  AllPortsSameDT=off  OutDataTypeStr=boolean
  OR : Logic  Operator=OR  IconShape=distinctive  AllPortsSameDT=off  OutDataTypeStr=boolean
  PID Controller : slpidlib/PID Controller  Controller=I  Form=Parallel  TimeDomain=Discrete-time  UseExternalTs=off  SampleTime=SampleTime  IntegratorMethod=Forward Euler  FilterMethod=Forward Euler  ControllerParametersSource=internal  P=1  I=1  UseKiTs=off  D=0  N=100  UseFilter=on  TunerSelectOption=Transfer Function Based (PID Tuner App)  InitialConditionSource=internal  InitialConditionForIntegrator=0  InitialConditionForFilter=0  DifferentiatorICPrevScaledInput=0  ExternalReset=rising  TrackingMode=off  Kt=1  LimitOutput=on  SatLimitsSource=internal  UpperSaturationLimit=10  LowerSaturationLimit=0  LinearizeAsGain=on  AntiWindupMode=clamping  Kb=1  POutMin=[]  POutMax=[]  IOutMin=[]  IOutMax=[]  DOutMin=[]  DOutMax=[]  NOutMin=[]  NOutMax=[]  SumOutMin=[]  SumOutMax=[]  SaturationOutMin=[]  SaturationOutMax=[]  PParamMin=[]  PParamMax=[]  IParamMin=[]  IParamMax=[]  DParamMin=[]  DParamMax=[]  NParamMin=[]  NParamMax=[]  KbParamMin=[]  KbParamMax=[]  KtParamMin=[]  KtParamMax=[]  KbOutMin=[]  KbOutMax=[]  KtOutMin=[]  KtOutMax=[]  IntegratorOutMin=[]  IntegratorOutMax=[]  FilterOutMin=[]  FilterOutMax=[]  SumI1OutMin=[]  SumI1OutMax=[]  SumI2OutMin=[]  SumI2OutMax=[]  SumI3OutMin=[]  SumI3OutMax=[]  SumI4OutMin=[]  SumI4OutMax=[]  SumDOutMin=[]  SumDOutMax=[]  DifferentiatorOutMin=[]  DifferentiatorOutMax=[]  FilterDiffOutCoefMin=[]  FilterDiffOutCoefMax=[]  ReciprocalOutMin=[]  ReciprocalOutMax=[]  SumDenOutMin=[]  SumDenOutMax=[]  SumNumOutMin=[]  SumNumOutMax=[]  DivideOutMin=[]  DivideOutMax=[]  UdiffTsProdOutMin=[]  UdiffTsProdOutMax=[]  NTsProdOutMin=[]  NTsProdOutMax=[]  UintegralTsProdOutMin=[]  UintegralTsProdOutMax=[]  UngainTsProdOutMin=[]  UngainTsProdOutMax=[]  IntegratorContinuousStateAttributes=''  IntegratorStateMustResolveToSignalObject=off  IntegratorRTWStateStorageClass=Auto  FilterContinuousStateAttributes=''  FilterStateMustResolveToSignalObject=off  FilterRTWStateStorageClass=Auto  ParallelPVariant=Disabled  IdealPVariant=Disabled  IVariant=InternalParameters  DVariant=Disabled  IntegratorVariant=Discrete  SatVariant=Enabled  AWVariant=DiscClampingParallel  PCopyVariant=Disabled  TRVariant=Disabled  FdbkBlocksVariant=Forward  IdealPFdbkVariant=Disabled  SatFdbkVariant=Disabled  DerivativeFilterVariant=Disabled  NVariant=Disabled  NCopyVariant=Disabled_SignalSpec  FilterICVariant=Disabled  IntegratorICVariant=InternalICs  ExternalResetVariant=ExternalReset  TRSumVariant=Passthrough  SumFdbkVariant=Disabled  SumVariant=Passthrough_I  TsampFilterVariant=InternalTs  TsampNgainVariant=Passthrough  TsampIntegralVariant=Passthrough  ExternalSaturationOutDataTypeStr=Inherit: Same as second input  aMode=0
  Relay1 : Relay  OnSwitchValue=13.8  OffSwitchValue=10.2  OutDataTypeStr=boolean
  Relay2 : Relay  OnSwitchValue=0.8  OffSwitchValue=0.2  OutDataTypeStr=boolean
  Relay3 : Relay  OnSwitchValue=9.95  OffSwitchValue=9.6  OnOutputValue=-3  OutDataTypeStr=single
  Sum : Sum  Inputs=|+-
  Sum1 : Sum
  Sum2 : Sum  Inputs=++++
  Alt_reset : Outport
  Pos_reset : Outport  Port=2
  All_reset : Outport  Port=3
  wires:
  Arm/1 -> Compare To Constant3/1
  Mode/1 -> Compare To Constant1/1
  Compare To Constant3/1 -> Data Type Conversion/1
  Compare To Constant1/1 -> NOT/1, Data Type Conversion1/1
  Data Type Conversion/1 -> Gain/1
  Sum2/1 -> Relay1/1
  Throttle/1 -> Compare To Constant4/1, Compare To Constant2/1
  Compare To Constant2/1 -> PID Controller/2, Data Type Conversion2/1
  Data Type Conversion2/1 -> Gain2/1
  Relay1/1 -> Alt_reset/1, OR/1
  Type/1 -> Data Type Conversion3/1
  Data Type Conversion3/1 -> Gain5/1
  Gain5/1 -> Sum1/2
  Gain/1 -> Sum2/1
  Data Type Conversion1/1 -> Gain1/1
  Compare To Constant4/1 -> AND/1
  Compare To Constant5/1 -> AND/2
  AND/1 -> Data Type Conversion4/1
  Data Type Conversion4/1 -> Gain3/1
  Constant/1 -> Sum/2
  PID Controller/1 -> Relay3/1
  Sum/1 -> PID Controller/1
  Gain1/1 -> Sum2/2
  Gain2/1 -> Sum2/3
  Relay3/1 -> Sum2/4
  Relay2/1 -> Pos_reset/1, OR/2
  OR/1 -> All_reset/1
  Vz/1 -> Gain4/1
  Gain4/1 -> Compare To Constant5/1
  Gain3/1 -> Sum/1
  NOT/1 -> Data Type Conversion5/1
  Data Type Conversion5/1 -> Gain6/1
  Gain6/1 -> Sum1/1
  Sum1/1 -> Relay2/1

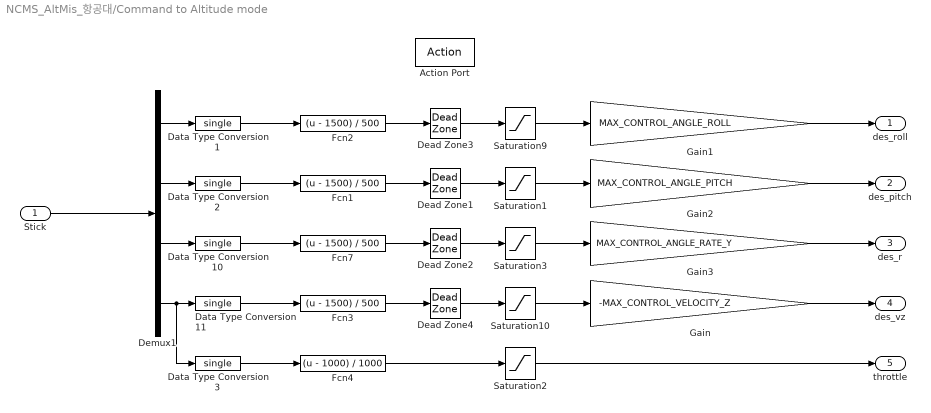
== system NCMS_AltMis_항공대/Command to Altitude mode ==
  Stick : Inport
  Action Port : ActionPort  InitializeStates=reset  ActionPortLabel=if(u1 < 1800)
  Data Type Conversion{1..3,10..11} (5 alike) : DataTypeConversion  OutDataTypeStr=single  SaturateOnIntegerOverflow=off  RndMeth=Floor
  Dead Zone1 : DeadZone  LowerValue=-0.001  UpperValue=0.001
  Dead Zone2 : DeadZone  LowerValue=-0.005  UpperValue=0.005
  Dead Zone3 : DeadZone  LowerValue=-0.003  UpperValue=0.003
  Dead Zone4 : DeadZone  LowerValue=-0.03  UpperValue=0.03
  Demux1 : Demux
  Fcn{1..3,7} (4 alike) : Fcn  Expr=(u - 1500) / 500
  Fcn4 : Fcn  Expr=(u - 1000) / 1000
  Gain : Gain  Gain=-MAX_CONTROL_VELOCITY_Z
  Gain1 : Gain  Gain=MAX_CONTROL_ANGLE_ROLL
  Gain2 : Gain  Gain=MAX_CONTROL_ANGLE_PITCH
  Gain3 : Gain  Gain=MAX_CONTROL_ANGLE_RATE_Y
  Saturation{1,3,9..10} (4 alike) : Saturate  UpperLimit=1  LowerLimit=-1
  Saturation2 : Saturate  UpperLimit=1  LowerLimit=0
  des_roll : Outport
  des_pitch : Outport  Port=2
  des_r : Outport  Port=3
  des_vz : Outport  Port=4
  throttle : Outport  Port=5
  wires:
  Fcn3/1 -> Dead Zone4/1
  Saturation10/1 -> Gain/1
  Gain1/1 -> des_roll/1
  Fcn1/1 -> Dead Zone1/1
  Data Type Conversion1/1 -> Fcn2/1
  Gain2/1 -> des_pitch/1
  Saturation1/1 -> Gain2/1
  Data Type Conversion11/1 -> Fcn3/1
  Dead Zone4/1 -> Saturation10/1
  Gain3/1 -> des_r/1
  Demux1/1 -> Data Type Conversion1/1
  Dead Zone1/1 -> Saturation1/1
  Saturation9/1 -> Gain1/1
  Saturation3/1 -> Gain3/1
  Demux1/4 -> Data Type Conversion3/1, Data Type Conversion11/1
  Data Type Conversion10/1 -> Fcn7/1
  Fcn2/1 -> Dead Zone3/1
  Stick/1 -> Demux1/1
  Demux1/2 -> Data Type Conversion2/1
  Dead Zone3/1 -> Saturation9/1
  Dead Zone2/1 -> Saturation3/1
  Fcn7/1 -> Dead Zone2/1
  Data Type Conversion2/1 -> Fcn1/1
  Demux1/3 -> Data Type Conversion10/1
  Data Type Conversion3/1 -> Fcn4/1
  Fcn4/1 -> Saturation2/1
  Saturation2/1 -> throttle/1
  Gain/1 -> des_vz/1

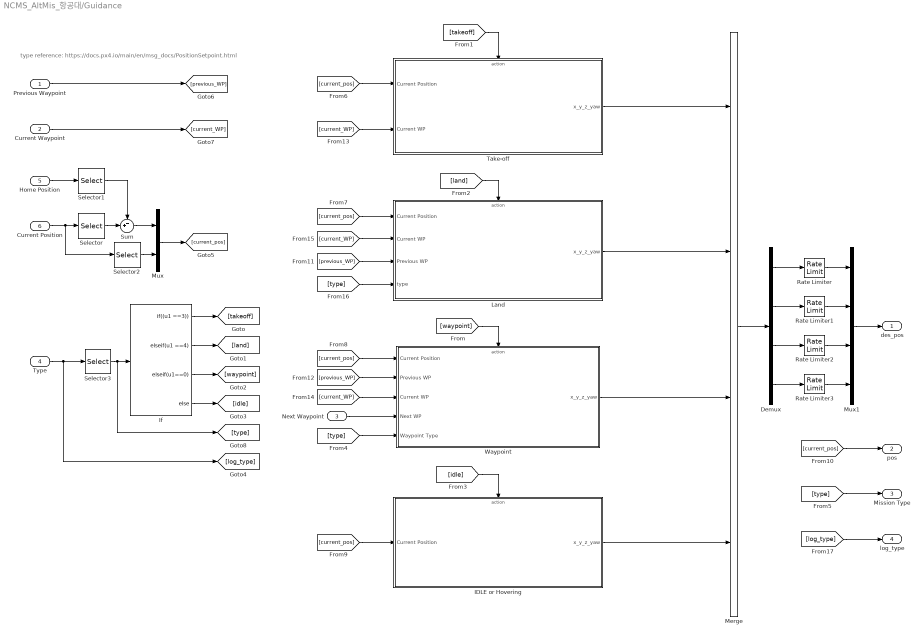
== system NCMS_AltMis_항공대/Guidance ==
  note: type reference: https://docs.px4.io/main/en/msg_docs/PositionSetpoint.html
  Previous Waypoint : Inport
  Current Waypoint : Inport  Port=2
  Next Waypoint : Inport  Port=3
  Type : Inport  Port=4
  Home Position : Inport  Port=5
  Current Position : Inport  Port=6
  Demux : Demux
  IDLE or Hovering : Subsystem  TreatAsAtomicUnit=on
  If : If  IfExpression=(u1 ==3)  ElseIfExpressions=u1 ==4, u1==0
  Land : Subsystem  TreatAsAtomicUnit=on
  Merge : Merge  Inputs=4
  Mux : Mux  Inputs=[3 1]
  Mux1 : Mux
  Rate Limiter : RateLimiter  RisingSlewLimit=MAX_CONTROL_VELOCITY_XY  FallingSlewLimit=-MAX_CONTROL_VELOCITY_XY  SampleTimeMode=inherited
  Rate Limiter1 : RateLimiter  RisingSlewLimit=MAX_CONTROL_VELOCITY_XY  FallingSlewLimit=-MAX_CONTROL_VELOCITY_XY  SampleTimeMode=inherited
  Rate Limiter2 : RateLimiter  RisingSlewLimit=MAX_CONTROL_VELOCITY_Z  FallingSlewLimit=-MAX_CONTROL_VELOCITY_Z  SampleTimeMode=inherited
  Rate Limiter3 : RateLimiter  RisingSlewLimit=MAX_CONTROL_ANGLE_RATE_Y  FallingSlewLimit=-MAX_CONTROL_ANGLE_RATE_Y  SampleTimeMode=inherited
  Selector : Selector  InputPortWidth=4  IndexOptions=Index vector (dialog)  Indices=[1 2 3]  OutputSizes=1
  Selector1 : Selector  InputPortWidth=4  IndexOptions=Index vector (dialog)  Indices=[1 2 3]  OutputSizes=1
  Selector2 : Selector  InputPortWidth=4  IndexOptions=Index vector (dialog)  Indices=4  OutputSizes=1
  Selector3 : Selector  InputPortWidth=3  IndexOptions=Index vector (dialog)  Indices=2  OutputSizes=1
  Sum : Sum  Inputs=-+|
  Take-off : Subsystem  TreatAsAtomicUnit=on
  Waypoint : Subsystem  TreatAsAtomicUnit=on
  des_pos : Outport
  pos : Outport  Port=2
  Mission Type : Outport  Port=3
  log_type : Outport  Port=4
  wires:
  Next Waypoint/1 -> Waypoint/4(Next WP)
  Mux/1 -> [current_pos]
  Type/1 -> [log_type], Selector3/1
  Take-off/1(x_y_z_yaw) -> Merge/1
  Land/1(x_y_z_yaw) -> Merge/2
  Waypoint/1(x_y_z_yaw) -> Merge/3
  IDLE or Hovering/1(x_y_z_yaw) -> Merge/4
  Current Position/1 -> Selector2/1, Selector/1
  Home Position/1 -> Selector1/1
  Selector1/1 -> Sum/1
  Sum/1 -> Mux/1
  Selector2/1 -> Mux/2
  [idle] -> IDLE or Hovering/Action
  [land] -> Land/Action
  [takeoff] -> Take-off/Action
  [waypoint] -> Waypoint/Action
  If/1 -> [takeoff]
  If/2 -> [land]
  If/3 -> [waypoint]
  If/4 -> [idle]
  [type] -> Waypoint/5(Waypoint Type)
  [type] -> Mission Type/1
  Selector/1 -> Sum/2
  [current_pos] -> pos/1
  [current_pos] -> Take-off/1(Current Position)
  [current_pos] -> Land/1(Current Position)
  [current_pos] -> Waypoint/1(Current Position)
  [current_pos] -> IDLE or Hovering/1(Current Position)
  Previous Waypoint/1 -> [previous_WP]
  [previous_WP] -> Land/3(Previous WP)
  [previous_WP] -> Waypoint/2(Previous WP)
  Current Waypoint/1 -> [current_WP]
  [current_WP] -> Take-off/2(Current WP)
  [current_WP] -> Land/2(Current WP)
  [current_WP] -> Waypoint/3(Current WP)
  Merge/1 -> Demux/1
  Demux/1 -> Rate Limiter/1
  Demux/2 -> Rate Limiter1/1
  Demux/3 -> Rate Limiter2/1
  Demux/4 -> Rate Limiter3/1
  Rate Limiter/1 -> Mux1/1
  Rate Limiter1/1 -> Mux1/2
  Rate Limiter2/1 -> Mux1/3
  Rate Limiter3/1 -> Mux1/4
  Mux1/1 -> des_pos/1
  Selector3/1 -> [type], If/1
  [type] -> Land/4(type)
  [log_type] -> log_type/1

== system NCMS_AltMis_항공대/Mixer ==
  tau_roll : Inport
  tau_pitch : Inport  Port=2
  tau_yaw : Inport  Port=3
  f : Inport  Port=4
  Throttle : Inport  Port=5
  Mode : Inport  Port=6
  Alt_reset : Inport  Port=7
  Pos_reset : Inport  Port=8
  Compare To Constant3 : simulink/Logic and Bit Operations/Compare To Constant  relop=<  const=uint16(1800)  OutDataTypeStr=boolean
  Constant : Constant  Value=THR_IDLE  OutDataTypeStr=single
  If : If  NumInputs=3  IfExpression=(u1 == 1)&(u2 == 0)  ElseIfExpressions=(u1 ~= 1)&(u3 == 0)
  If Action Subsystem : Subsystem  TreatAsAtomicUnit=on
  If Action Subsystem1 : Subsystem  TreatAsAtomicUnit=on
  If Action Subsystem2 : Subsystem  TreatAsAtomicUnit=on
  Merge : Merge  Inputs=3
  Output_Limits1 : Saturate  UpperLimit=2000  LowerLimit=1200  OutDataTypeStr=uint16
  Mn : Outport
  wires:
  Mode/1 -> Compare To Constant3/1
  Alt_reset/1 -> If/2
  Pos_reset/1 -> If/3
  f/1 -> If Action Subsystem2/4(Thrust)
  Merge/1 -> Output_Limits1/1
  If/1 -> If Action Subsystem/Action
  tau_roll/1 -> If Action Subsystem2/1(Roll), If Action Subsystem1/1(Roll), If Action Subsystem/1(Roll)
  tau_pitch/1 -> If Action Subsystem2/2(Pitch), If Action Subsystem1/2(Pitch), If Action Subsystem/2(Pitch)
  tau_yaw/1 -> If Action Subsystem/3(Yaw), If Action Subsystem1/3(Yaw), If Action Subsystem2/3(Yaw)
  Throttle/1 -> If Action Subsystem/4(Thrust)
  If/2 -> If Action Subsystem1/Action
  Constant/1 -> If Action Subsystem1/4(Thrust)
  If/3 -> If Action Subsystem2/Action
  If Action Subsystem/1(Out1) -> Merge/1
  If Action Subsystem1/1(Out1) -> Merge/2
  If Action Subsystem2/1(Out1) -> Merge/3
  Compare To Constant3/1 -> If/1
  Output_Limits1/1 -> Mn/1

== system NCMS_AltMis_항공대/Postion Controller ==
  des_pos : Inport
  pos : Inport  Port=2
  vel : Inport  Port=3
  Pos_reset : Inport  Port=4
  Action Port : ActionPort  InitializeStates=reset  ActionPortLabel=else
  Demux : Demux
  Demux1 : Demux
  Demux2 : Demux  Outputs=3
  Position Controller : Subsystem
      settings: PortSchema="{\"entries\":[{\"content\":{\"sides\":[{\"content\":{\"connectorIds\":[\"In1\",\"In2\",\"In3\",\"In4\",\"In5\",\"In6\",\"In7\",\"In8\",\"In9\",\"In10\"]},\"type\":\"ConnectorPlacement.EquallySpacedRectSide\",\"uuid\":\"5bde12f8-959d-4edf-9b00-69b1c3e0ccd9\"},{\"content\":{\"connectorIds\":[\"Out1\",\"Out2\",\"Out3\",\"Out4\",\"Out5\"],\"side\":\"RIGHT\"},\"type\":\"ConnectorPlacement.EquallySpacedRectSide\",\"uuid\":\"6ee4afcd-5e59-4749-a6f3-cec7fc0963cb\"},{\"content\":{\"connectorIds\":[\"In11\"],\"side\":\"TOP\"},\"type\":\"ConnectorPlacement.EquallySpacedRectSide\",\"uuid\":\"fd5a4acc-2659-4eb5-b6a6-ae5db7fe0238\"}]},\"type\":\"ConnectorPlacement.EquallySpacedConnector\",\"uuid\":\"ee308163-0a0c-496a-b151-b7491420ab89\"}],\"packageUris\":[\"http://schema.mathworks.com/mf0/Connector/R2020b\"],\"version\":\"1.0\"}"
  Terminator : Terminator
  des_roll : Outport
  des_pitch : Outport  Port=2
  des_r : Outport  Port=3
  des_vz : Outport  Port=4
  log : Outport  Port=5
  wires:
  Demux/1 -> Position Controller/1(des_x)
  Demux/2 -> Position Controller/2(des_y)
  Demux/3 -> Position Controller/3(des_alt)
  des_pos/1 -> Demux/1
  Demux1/1 -> Position Controller/5(x)
  Demux1/2 -> Position Controller/6(y)
  Demux1/3 -> Position Controller/7(z)
  pos/1 -> Demux1/1
  Demux2/1 -> Position Controller/9(vx)
  Demux2/2 -> Position Controller/10(vy)
  Demux2/3 -> Terminator/1
  vel/1 -> Demux2/1
  Position Controller/2(des_pitch) -> des_pitch/1
  Position Controller/1(des_roll) -> des_roll/1
  Demux/4 -> Position Controller/4(des_yaw)
  Position Controller/4(des_vz) -> des_vz/1
  Demux1/4 -> Position Controller/8(yaw_angle)
  Pos_reset/1 -> Position Controller/11(reset_sig)
  Position Controller/3(des_r) -> des_r/1
  Position Controller/5(log) -> log/1

== system NCMS_AltMis_항공대/Read uORB ==
  Bus Selector : BusSelector  OutputSignals=x,y,z,yaw  OutputAsBus=on
  Bus Selector1 : BusSelector  OutputSignals=vx,vy,vz  OutputAsBus=on
  Data Type Conversion : DataTypeConversion  OutDataTypeStr=double  SaturateOnIntegerOverflow=off  RndMeth=Floor
  Data Type Conversion9 : DataTypeConversion  OutDataTypeStr=single  SaturateOnIntegerOverflow=off  RndMeth=Floor
  Gyroscope : px4Sensorslib/Gyroscope  uorbTimeStamp=off  BlockingMode=off  BlockTimeout=1e-3  sampleTime=SampleTime
      settings: SourceProductBaseCode=PX4AUTOPILOTS
  Mux : Mux  Inputs=3
  PX4 uORB Read : px4uORBlib/PX4 uORB Read  uORBTopic=vehicle_local_position  selectInstance=vehicle_local_position  SampleTime=SampleTime  BlockingMode=off  BlockTimeout=1e-3
      settings: SourceProductBaseCode=PX4AUTOPILOTS
  Terminator : Terminator
  Terminator5 : Terminator
  Terminator7 : Terminator
  Vehicle Attitude : px4Sensorslib/Vehicle Attitude  rollRate=off  pitchRate=off  yawRate=off  quaternion=on  uorbTimeStamp=off  BlockingMode=off  BlockTimeout=0.001  sampleTime=SampleTime
      settings: SourceProductBaseCode=PX4AUTOPILOTS
  Pos : Outport
  Vel : Outport  Port=2
  Quat : Outport  Port=3
  pqr : Outport  Port=4
  wires:
  Vehicle Attitude/1 -> Terminator5/1
  Gyroscope/4 -> Mux/3
  Gyroscope/3 -> Mux/2
  Gyroscope/2 -> Mux/1
  Gyroscope/1 -> Terminator7/1
  PX4 uORB Read/1 -> Terminator/1
  PX4 uORB Read/2 -> Bus Selector1/1, Bus Selector/1
  Mux/1 -> pqr/1
  Vehicle Attitude/2 -> Quat/1
  Bus Selector1/1 -> Data Type Conversion9/1
  Bus Selector/1 -> Data Type Conversion/1
  Data Type Conversion/1 -> Pos/1
  Data Type Conversion9/1 -> Vel/1

== system NCMS_AltMis_항공대/Read wapoints from Mission in QGC ==
  Bus Selector : BusSelector  OutputSignals=previous,current,next
  Convert LLA to NED : MATLAB Function  TreatAsAtomicUnit=on
  PX4 uORB Read : px4uORBlib/PX4 uORB Read  uORBTopic=home_position  selectInstance=home_position  SampleTime=SampleTime  BlockingMode=off  BlockTimeout=1e-3
      settings: SourceProductBaseCode=PX4AUTOPILOTS
  PX4 uORB Read1 : px4uORBlib/PX4 uORB Read  uORBTopic=position_setpoint_triplet  selectInstance=position_setpoint_triplet  SampleTime=SampleTime  BlockingMode=off  BlockTimeout=1e-3
      settings: SourceProductBaseCode=PX4AUTOPILOTS
  Subsystem : Subsystem
  Terminator : Terminator
  Terminator1 : Terminator
  Previous Waypoint : Outport
  Current Waypoint : Outport  Port=2
  Next Waypoint : Outport  Port=3
  Type : Outport  Port=4
  Home Position : Outport  Port=5
  wires:
  Bus Selector/1 -> Subsystem/1(previousSetpoint_msg)  "<previous>"
  Bus Selector/2 -> Subsystem/2(currentSetpoint_msg)  "<current>"
  Subsystem/3(nextSetpoint) -> Convert LLA to NED/3(nextSetpoint)
  Subsystem/2(currentSetpoint) -> Convert LLA to NED/2(currentSetpoint)
  PX4 uORB Read1/1 -> Terminator1/1
  Bus Selector/3 -> Subsystem/3(nextSetpoint_msg)  "<next>"
  Convert LLA to NED/3(next) -> Next Waypoint/1
  Subsystem/4(homePostion_LLA) -> Convert LLA to NED/4(homePosition)
  Convert LLA to NED/1(previous) -> Previous Waypoint/1
  PX4 uORB Read1/2 -> Bus Selector/1
  Subsystem/1(previousSetpoint) -> Convert LLA to NED/1(previousSetpoint)
  PX4 uORB Read/1 -> Terminator/1
  PX4 uORB Read/2 -> Subsystem/4(homePosition_msg)
  Subsystem/5(homePostion_local) -> Home Position/1
  Convert LLA to NED/2(current) -> Current Waypoint/1
  Convert LLA to NED/4(type) -> Type/1

== system NCMS_AltMis_항공대/Remote Control ==
  Mux3 : Mux
  Radio Control Transmitter : px4Sensorslib/Radio Control Transmitter  channel1=on  channel2=on  channel3=on  channel4=on  channel5=on  channel6=on  channel7=off  channel8=off  channel_count=off  rssi=off  rc_input_source=off  timestamp_last_signal=off  time_stamp=off  sampleTime=SampleTime  BlockingMode=off  BlockTimeout=5
      settings: SourceProductBaseCode=PX4AUTOPILOTS
  Terminator1 : Terminator
  Arm : Outport
  Mode : Outport  Port=2
  Throttle : Outport  Port=3
  Stick : Outport  Port=4
  wires:
  Radio Control Transmitter/5 -> Throttle/1, Mux3/4  "throttle, des_vz"
  Radio Control Transmitter/6 -> Arm/1  "arm_signal"
  Radio Control Transmitter/4 -> Mux3/3  "des_r"
  Radio Control Transmitter/2 -> Mux3/1  "des_R"
  Mux3/1 -> Stick/1
  Radio Control Transmitter/1 -> Terminator1/1
  Radio Control Transmitter/3 -> Mux3/2  "des_P"
  Radio Control Transmitter/7 -> Mode/1  "mode_signal"

== system NCMS_AltMis_항공대/Subsystem1 ==
  arm : Inport
  mode : Inport  Port=2
  type : Inport  Port=3
  PWMout : Inport  Port=4
  Data Type Conversion : DataTypeConversion  OutDataTypeStr=uint16  SaturateOnIntegerOverflow=off  RndMeth=Floor
  Demux1 : Demux  Outputs=3
  Demux10 : Demux
  Mux1 : Mux  Inputs=9
  To Workspace17 : ToWorkspace  VariableName=log_uint16  SaveFormat=Structure With Time  SampleTime=SampleTime
      settings: Save2DSignal=2-D array (concatenate along first dimension)
  wires:
  Mux1/1 -> To Workspace17/1
  PWMout/1 -> Demux10/1
  type/1 -> Data Type Conversion/1
  arm/1 -> Mux1/1
  mode/1 -> Mux1/2
  Demux1/3 -> Mux1/5  "next"
  Demux1/2 -> Mux1/4  "current"
  Demux1/1 -> Mux1/3  "previous"
  Data Type Conversion/1 -> Demux1/1  "type"
  Demux10/1 -> Mux1/6  "M1"
  Demux10/2 -> Mux1/7  "M2"
  Demux10/3 -> Mux1/8  "M3"
  Demux10/4 -> Mux1/9  "M4"
